simulink model "FrankSensingDiscreteEKF"  (R2025a)
settings: Solver=FixedStepAuto  StartTime=0.0  StopTime=150  FixedStep=.001  RelTol=1e-3
model workspace (MAT data in the model file):
  GPSvehyUpdate = 0
libraries: simulink x1
(part 2 of 2)

== matlab function FrankSensingDiscreteEKF/MATLAB Function1 ==
  data: P output; VYmeas input; X output; VXmeas input; rmeas input; Axmeas input; Xcov input; Ycov input; Ppri input; Xpri input; startflag input; SA input; res output; fk output; Rbiaspri output; Abiaspri output
function [P,X,res,fk,Rbiaspri,Abiaspri] = fcn(VYmeas,VXmeas,rmeas,Axmeas,Xcov,Ycov,Ppri,Xpri, startflag, SA)

a = .3036;
b = .2484;
B = 8.45;
C = 1.6;
D = 73.1580;
E = 1;
Iz = 1;
Mv = 15.7;
delta = SA;
Ts = 0.001;

rvar = .01;
Axvar = .001;


Rk = [Ycov    0    0   0;... 
      0        Xcov    0   0;...
      0        0        rvar    0
      0        0        0       Axvar];  %Measurement noise covariance matrix


Qk = [.02     0      0       0       0       0       0;...
      0      .02      0       0      0       0       0;...
      0      0       .01      0      0       0       0;...
      0      0      0       .01     0       0       0;...
      0      0      0       0       .0001     0       0;...
      0      0      0       0       0       .0001     0;...
      0      0      0       0       0       0       .0001]; % process noise covariance matrix

zk = [VYmeas; VXmeas; rmeas; Axmeas];

% Startup Initialization

if startflag == 0

    Ppredict = [.1     0      0       0       0       0       0;...
      0      .1      0       0      0       0       0;...
      0      0       .1      0      0       0       0;...
      0      0      0       .1     0       0       0;...
      0      0      0       0       .001     0       0;...
      0      0      0       0       0       .001     0;...
      0      0      0       0       0       0       .001];

    
    Xpri = [0.5;-1.9;-.49;0;0.34;-.022;-0.2];
      
else

    Ppredict = Ppri;
end

%Predict:

Vypri = Xpri(1);
Vxpri = Xpri(2);
rpri = Xpri(3);
Psipri = Xpri(4);
Axpri = Xpri(5);
Rbiaspri = Xpri(6);
Abiaspri = Xpri(7);

fk =  LittleF(Abiaspri,Axpri,B,C,D,E,Iz,Mv,Psipri,Rbiaspri,Ts,Vxpri,Vypri,a,b,delta,rpri);

% fk =    [Vypri - Ts*(Vxpri*rpri - (D*sin(C*atan(B*atan((Vypri + b*(Rbiaspri + rpri))/Vxpri) + E*(atan(B*atan((Vypri + b*(Rbiaspri + rpri))/Vxpri)) - B*atan((Vypri + b*(Rbiaspri + rpri))/Vxpri)))) + D*sin(C*atan(E*(atan(B*(delta + atan((Vypri - a*(Rbiaspri + rpri))/Vxpri))) - B*(delta + atan((Vypri - a*(Rbiaspri + rpri))/Vxpri))) + B*(delta + atan((Vypri - a*(Rbiaspri + rpri))/Vxpri))))*cos(delta))/Mv);...
%                                                                                                                                                                                                                                                                                                                                                                      Vxpri + Ts*(Abiaspri + Axpri - Vypri*rpri);...
%     Rbiaspri + rpri - (Ts*(D*b*sin(C*atan(B*atan((Vypri + b*(Rbiaspri + rpri))/Vxpri) + E*(atan(B*atan((Vypri + b*(Rbiaspri + rpri))/Vxpri)) - B*atan((Vypri + b*(Rbiaspri + rpri))/Vxpri)))) - D*a*sin(C*atan(E*(atan(B*(delta + atan((Vypri - a*(Rbiaspri + rpri))/Vxpri))) - B*(delta + atan((Vypri - a*(Rbiaspri + rpri))/Vxpri))) + B*(delta + atan((Vypri - a*(Rbiaspri + rpri))/Vxpri))))*cos(delta)))/Iz;...
%                                                                                                                                                                                                                                                                                                                                                                                   Psipri + Ts*(Rbiaspri + rpri);...
%                                                                                                                                                                                                                                                                                                                                                                                              Abiaspri + Axpri;...
%                                                                                                                                                                                                                                                                                                                                                                                                         Rbiaspri;...
%                                                                                                                                                                                                                                                                                                                                                                                                     Abiaspri];
% 
% 
% 
% 
Fk = BigF(B,C,D,E,Iz,Mv,Rbiaspri,Ts,Vxpri,Vypri,a,b,delta,rpri)

% Fk = [1 - (Ts*((C*D*cos(C*atan(B*atan((Vypri + b*(Rbiaspri + rpri))/Vxpri) + E*(atan(B*atan((Vypri + b*(Rbiaspri + rpri))/Vxpri)) - B*atan((Vypri + b*(Rbiaspri + rpri))/Vxpri))))*(E*(B/(Vxpri*((Vypri + b*(Rbiaspri + rpri))^2/Vxpri^2 + 1)) - B/(Vxpri*((Vypri + b*(Rbiaspri + rpri))^2/Vxpri^2 + 1)*(B^2*atan((Vypri + b*(Rbiaspri + rpri))/Vxpri)^2 + 1))) - B/(Vxpri*((Vypri + b*(Rbiaspri + rpri))^2/Vxpri^2 + 1))))/((B*atan((Vypri + b*(Rbiaspri + rpri))/Vxpri) + E*(atan(B*atan((Vypri + b*(Rbiaspri + rpri))/Vxpri)) - B*atan((Vypri + b*(Rbiaspri + rpri))/Vxpri)))^2 + 1) + (C*D*cos(C*atan(E*(atan(B*(delta + atan((Vypri - a*(Rbiaspri + rpri))/Vxpri))) - B*(delta + atan((Vypri - a*(Rbiaspri + rpri))/Vxpri))) + B*(delta + atan((Vypri - a*(Rbiaspri + rpri))/Vxpri))))*cos(delta)*(E*(B/(Vxpri*((Vypri - a*(Rbiaspri + rpri))^2/Vxpri^2 + 1)) - B/(Vxpri*((Vypri - a*(Rbiaspri + rpri))^2/Vxpri^2 + 1)*(B^2*(delta + atan((Vypri - a*(Rbiaspri + rpri))/Vxpri))^2 + 1))) - B/(Vxpri*((Vypri - a*(Rbiaspri + rpri))^2/Vxpri^2 + 1))))/((E*(atan(B*(delta + atan((Vypri - a*(Rbiaspri + rpri))/Vxpri))) - B*(delta + atan((Vypri - a*(Rbiaspri + rpri))/Vxpri))) + B*(delta + atan((Vypri - a*(Rbiaspri + rpri))/Vxpri)))^2 + 1)))/Mv, -Ts*(rpri - ((C*D*cos(C*atan(B*atan((Vypri + b*(Rbiaspri + rpri))/Vxpri) + E*(atan(B*atan((Vypri + b*(Rbiaspri + rpri))/Vxpri)) - B*atan((Vypri + b*(Rbiaspri + rpri))/Vxpri))))*(E*((B*(Vypri + b*(Rbiaspri + rpri)))/(Vxpri^2*((Vypri + b*(Rbiaspri + rpri))^2/Vxpri^2 + 1)) - (B*(Vypri + b*(Rbiaspri + rpri)))/(Vxpri^2*((Vypri + b*(Rbiaspri + rpri))^2/Vxpri^2 + 1)*(B^2*atan((Vypri + b*(Rbiaspri + rpri))/Vxpri)^2 + 1))) - (B*(Vypri + b*(Rbiaspri + rpri)))/(Vxpri^2*((Vypri + b*(Rbiaspri + rpri))^2/Vxpri^2 + 1))))/((B*atan((Vypri + b*(Rbiaspri + rpri))/Vxpri) + E*(atan(B*atan((Vypri + b*(Rbiaspri + rpri))/Vxpri)) - B*atan((Vypri + b*(Rbiaspri + rpri))/Vxpri)))^2 + 1) + (C*D*cos(C*atan(E*(atan(B*(delta + atan((Vypri - a*(Rbiaspri + rpri))/Vxpri))) - B*(delta + atan((Vypri - a*(Rbiaspri + rpri))/Vxpri))) + B*(delta + atan((Vypri - a*(Rbiaspri + rpri))/Vxpri))))*cos(delta)*(E*((B*(Vypri - a*(Rbiaspri + rpri)))/(Vxpri^2*((Vypri - a*(Rbiaspri + rpri))^2/Vxpri^2 + 1)) - (B*(Vypri - a*(Rbiaspri + rpri)))/(Vxpri^2*((Vypri - a*(Rbiaspri + rpri))^2/Vxpri^2 + 1)*(B^2*(delta + atan((Vypri - a*(Rbiaspri + rpri))/Vxpri))^2 + 1))) - (B*(Vypri - a*(Rbiaspri + rpri)))/(Vxpri^2*((Vypri - a*(Rbiaspri + rpri))^2/Vxpri^2 + 1))))/((E*(atan(B*(delta + atan((Vypri - a*(Rbiaspri + rpri))/Vxpri))) - B*(delta + atan((Vypri - a*(Rbiaspri + rpri))/Vxpri))) + B*(delta + atan((Vypri - a*(Rbiaspri + rpri))/Vxpri)))^2 + 1))/Mv), -Ts*(Vxpri + ((C*D*cos(C*atan(B*atan((Vypri + b*(Rbiaspri + rpri))/Vxpri) + E*(atan(B*atan((Vypri + b*(Rbiaspri + rpri))/Vxpri)) - B*atan((Vypri + b*(Rbiaspri + rpri))/Vxpri))))*(E*((B*b)/(Vxpri*((Vypri + b*(Rbiaspri + rpri))^2/Vxpri^2 + 1)) - (B*b)/(Vxpri*((Vypri + b*(Rbiaspri + rpri))^2/Vxpri^2 + 1)*(B^2*atan((Vypri + b*(Rbiaspri + rpri))/Vxpri)^2 + 1))) - (B*b)/(Vxpri*((Vypri + b*(Rbiaspri + rpri))^2/Vxpri^2 + 1))))/((B*atan((Vypri + b*(Rbiaspri + rpri))/Vxpri) + E*(atan(B*atan((Vypri + b*(Rbiaspri + rpri))/Vxpri)) - B*atan((Vypri + b*(Rbiaspri + rpri))/Vxpri)))^2 + 1) - (C*D*cos(C*atan(E*(atan(B*(delta + atan((Vypri - a*(Rbiaspri + rpri))/Vxpri))) - B*(delta + atan((Vypri - a*(Rbiaspri + rpri))/Vxpri))) + B*(delta + atan((Vypri - a*(Rbiaspri + rpri))/Vxpri))))*cos(delta)*(E*((B*a)/(Vxpri*((Vypri - a*(Rbiaspri + rpri))^2/Vxpri^2 + 1)) - (B*a)/(Vxpri*((Vypri - a*(Rbiaspri + rpri))^2/Vxpri^2 + 1)*(B^2*(delta + atan((Vypri - a*(Rbiaspri + rpri))/Vxpri))^2 + 1))) - (B*a)/(Vxpri*((Vypri - a*(Rbiaspri + rpri))^2/Vxpri^2 + 1))))/((E*(atan(B*(delta + atan((Vypri - a*(Rbiaspri + rpri))/Vxpri))) - B*(delta + atan((Vypri - a*(Rbiaspri + rpri))/Vxpri))) + B*(delta + atan((Vypri - a*(Rbiaspri + rpri))/Vxpri)))^2 + 1))/Mv), 0,  0,        -(Ts*((C*D*cos(C*atan(B*atan((Vypri + b*(Rbiaspri + rpri))/Vxpri) + E*(atan(B*atan((Vypri + b*(Rbiaspri + rpri))/Vxpri)) - B*atan((Vypri + b*(Rbiaspri + rpri))/Vxpri))))*(E*((B*b)/(Vxpri*((Vypri + b*(Rbiaspri + rpri))^2/Vxpri^2 + 1)) - (B*b)/(Vxpri*((Vypri + b*(Rbiaspri + rpri))^2/Vxpri^2 + 1)*(B^2*atan((Vypri + b*(Rbiaspri + rpri))/Vxpri)^2 + 1))) - (B*b)/(Vxpri*((Vypri + b*(Rbiaspri + rpri))^2/Vxpri^2 + 1))))/((B*atan((Vypri + b*(Rbiaspri + rpri))/Vxpri) + E*(atan(B*atan((Vypri + b*(Rbiaspri + rpri))/Vxpri)) - B*atan((Vypri + b*(Rbiaspri + rpri))/Vxpri)))^2 + 1) - (C*D*cos(C*atan(E*(atan(B*(delta + atan((Vypri - a*(Rbiaspri + rpri))/Vxpri))) - B*(delta + atan((Vypri - a*(Rbiaspri + rpri))/Vxpri))) + B*(delta + atan((Vypri - a*(Rbiaspri + rpri))/Vxpri))))*cos(delta)*(E*((B*a)/(Vxpri*((Vypri - a*(Rbiaspri + rpri))^2/Vxpri^2 + 1)) - (B*a)/(Vxpri*((Vypri - a*(Rbiaspri + rpri))^2/Vxpri^2 + 1)*(B^2*(delta + atan((Vypri - a*(Rbiaspri + rpri))/Vxpri))^2 + 1))) - (B*a)/(Vxpri*((Vypri - a*(Rbiaspri + rpri))^2/Vxpri^2 + 1))))/((E*(atan(B*(delta + atan((Vypri - a*(Rbiaspri + rpri))/Vxpri))) - B*(delta + atan((Vypri - a*(Rbiaspri + rpri))/Vxpri))) + B*(delta + atan((Vypri - a*(Rbiaspri + rpri))/Vxpri)))^2 + 1)))/Mv,  0;...
%                                                                                                                                                                                                                                                                                                                                                                                                                                                                                                                                                                                                                                                                                                                                                                                                                                                                                                                                                                                                                                                                                                                                                                                                                                               -Ts*rpri,                                                                                                                                                                                                                                                                                                                                                                                                                                                                                                                                                                                                                                                                                                                                                                                                                                                                                                                                                                                                                                                                                                                                                                                                                                                                                                                                                                                                                                                                  1,                                                                                                                                                                                                                                                                                                                                                                                                                                                                                                                                                                                                                                                                                                                                                                                                                                                                                                                                                                                                                                                                                                                                                                                                                                                                       -Ts*Vypri, 0, Ts,                                                                                                                                                                                                                                                                                                                                                                                                                                                                                                                                                                                                                                                                                                                                                                                                                                                                                                                                                                                                                                                                                                                                                                                                                                                                              0, Ts;...
%     (Ts*((C*D*b*cos(C*atan(B*atan((Vypri + b*(Rbiaspri + rpri))/Vxpri) + E*(atan(B*atan((Vypri + b*(Rbiaspri + rpri))/Vxpri)) - B*atan((Vypri + b*(Rbiaspri + rpri))/Vxpri))))*(E*(B/(Vxpri*((Vypri + b*(Rbiaspri + rpri))^2/Vxpri^2 + 1)) - B/(Vxpri*((Vypri + b*(Rbiaspri + rpri))^2/Vxpri^2 + 1)*(B^2*atan((Vypri + b*(Rbiaspri + rpri))/Vxpri)^2 + 1))) - B/(Vxpri*((Vypri + b*(Rbiaspri + rpri))^2/Vxpri^2 + 1))))/((B*atan((Vypri + b*(Rbiaspri + rpri))/Vxpri) + E*(atan(B*atan((Vypri + b*(Rbiaspri + rpri))/Vxpri)) - B*atan((Vypri + b*(Rbiaspri + rpri))/Vxpri)))^2 + 1) - (C*D*a*cos(C*atan(E*(atan(B*(delta + atan((Vypri - a*(Rbiaspri + rpri))/Vxpri))) - B*(delta + atan((Vypri - a*(Rbiaspri + rpri))/Vxpri))) + B*(delta + atan((Vypri - a*(Rbiaspri + rpri))/Vxpri))))*cos(delta)*(E*(B/(Vxpri*((Vypri - a*(Rbiaspri + rpri))^2/Vxpri^2 + 1)) - B/(Vxpri*((Vypri - a*(Rbiaspri + rpri))^2/Vxpri^2 + 1)*(B^2*(delta + atan((Vypri - a*(Rbiaspri + rpri))/Vxpri))^2 + 1))) - B/(Vxpri*((Vypri - a*(Rbiaspri + rpri))^2/Vxpri^2 + 1))))/((E*(atan(B*(delta + atan((Vypri - a*(Rbiaspri + rpri))/Vxpri))) - B*(delta + atan((Vypri - a*(Rbiaspri + rpri))/Vxpri))) + B*(delta + atan((Vypri - a*(Rbiaspri + rpri))/Vxpri)))^2 + 1)))/Iz,    -(Ts*((C*D*b*cos(C*atan(B*atan((Vypri + b*(Rbiaspri + rpri))/Vxpri) + E*(atan(B*atan((Vypri + b*(Rbiaspri + rpri))/Vxpri)) - B*atan((Vypri + b*(Rbiaspri + rpri))/Vxpri))))*(E*((B*(Vypri + b*(Rbiaspri + rpri)))/(Vxpri^2*((Vypri + b*(Rbiaspri + rpri))^2/Vxpri^2 + 1)) - (B*(Vypri + b*(Rbiaspri + rpri)))/(Vxpri^2*((Vypri + b*(Rbiaspri + rpri))^2/Vxpri^2 + 1)*(B^2*atan((Vypri + b*(Rbiaspri + rpri))/Vxpri)^2 + 1))) - (B*(Vypri + b*(Rbiaspri + rpri)))/(Vxpri^2*((Vypri + b*(Rbiaspri + rpri))^2/Vxpri^2 + 1))))/((B*atan((Vypri + b*(Rbiaspri + rpri))/Vxpri) + E*(atan(B*atan((Vypri + b*(Rbiaspri + rpri))/Vxpri)) - B*atan((Vypri + b*(Rbiaspri + rpri))/Vxpri)))^2 + 1) - (C*D*a*cos(C*atan(E*(atan(B*(delta + atan((Vypri - a*(Rbiaspri + rpri))/Vxpri))) - B*(delta + atan((Vypri - a*(Rbiaspri + rpri))/Vxpri))) + B*(delta + atan((Vypri - a*(Rbiaspri + rpri))/Vxpri))))*cos(delta)*(E*((B*(Vypri - a*(Rbiaspri + rpri)))/(Vxpri^2*((Vypri - a*(Rbiaspri + rpri))^2/Vxpri^2 + 1)) - (B*(Vypri - a*(Rbiaspri + rpri)))/(Vxpri^2*((Vypri - a*(Rbiaspri + rpri))^2/Vxpri^2 + 1)*(B^2*(delta + atan((Vypri - a*(Rbiaspri + rpri))/Vxpri))^2 + 1))) - (B*(Vypri - a*(Rbiaspri + rpri)))/(Vxpri^2*((Vypri - a*(Rbiaspri + rpri))^2/Vxpri^2 + 1))))/((E*(atan(B*(delta + atan((Vypri - a*(Rbiaspri + rpri))/Vxpri))) - B*(delta + atan((Vypri - a*(Rbiaspri + rpri))/Vxpri))) + B*(delta + atan((Vypri - a*(Rbiaspri + rpri))/Vxpri)))^2 + 1)))/Iz,  (Ts*((C*D*b*cos(C*atan(B*atan((Vypri + b*(Rbiaspri + rpri))/Vxpri) + E*(atan(B*atan((Vypri + b*(Rbiaspri + rpri))/Vxpri)) - B*atan((Vypri + b*(Rbiaspri + rpri))/Vxpri))))*(E*((B*b)/(Vxpri*((Vypri + b*(Rbiaspri + rpri))^2/Vxpri^2 + 1)) - (B*b)/(Vxpri*((Vypri + b*(Rbiaspri + rpri))^2/Vxpri^2 + 1)*(B^2*atan((Vypri + b*(Rbiaspri + rpri))/Vxpri)^2 + 1))) - (B*b)/(Vxpri*((Vypri + b*(Rbiaspri + rpri))^2/Vxpri^2 + 1))))/((B*atan((Vypri + b*(Rbiaspri + rpri))/Vxpri) + E*(atan(B*atan((Vypri + b*(Rbiaspri + rpri))/Vxpri)) - B*atan((Vypri + b*(Rbiaspri + rpri))/Vxpri)))^2 + 1) + (C*D*a*cos(C*atan(E*(atan(B*(delta + atan((Vypri - a*(Rbiaspri + rpri))/Vxpri))) - B*(delta + atan((Vypri - a*(Rbiaspri + rpri))/Vxpri))) + B*(delta + atan((Vypri - a*(Rbiaspri + rpri))/Vxpri))))*cos(delta)*(E*((B*a)/(Vxpri*((Vypri - a*(Rbiaspri + rpri))^2/Vxpri^2 + 1)) - (B*a)/(Vxpri*((Vypri - a*(Rbiaspri + rpri))^2/Vxpri^2 + 1)*(B^2*(delta + atan((Vypri - a*(Rbiaspri + rpri))/Vxpri))^2 + 1))) - (B*a)/(Vxpri*((Vypri - a*(Rbiaspri + rpri))^2/Vxpri^2 + 1))))/((E*(atan(B*(delta + atan((Vypri - a*(Rbiaspri + rpri))/Vxpri))) - B*(delta + atan((Vypri - a*(Rbiaspri + rpri))/Vxpri))) + B*(delta + atan((Vypri - a*(Rbiaspri + rpri))/Vxpri)))^2 + 1)))/Iz + 1, 0,  0, (Ts*((C*D*b*cos(C*atan(B*atan((Vypri + b*(Rbiaspri + rpri))/Vxpri) + E*(atan(B*atan((Vypri + b*(Rbiaspri + rpri))/Vxpri)) - B*atan((Vypri + b*(Rbiaspri + rpri))/Vxpri))))*(E*((B*b)/(Vxpri*((Vypri + b*(Rbiaspri + rpri))^2/Vxpri^2 + 1)) - (B*b)/(Vxpri*((Vypri + b*(Rbiaspri + rpri))^2/Vxpri^2 + 1)*(B^2*atan((Vypri + b*(Rbiaspri + rpri))/Vxpri)^2 + 1))) - (B*b)/(Vxpri*((Vypri + b*(Rbiaspri + rpri))^2/Vxpri^2 + 1))))/((B*atan((Vypri + b*(Rbiaspri + rpri))/Vxpri) + E*(atan(B*atan((Vypri + b*(Rbiaspri + rpri))/Vxpri)) - B*atan((Vypri + b*(Rbiaspri + rpri))/Vxpri)))^2 + 1) + (C*D*a*cos(C*atan(E*(atan(B*(delta + atan((Vypri - a*(Rbiaspri + rpri))/Vxpri))) - B*(delta + atan((Vypri - a*(Rbiaspri + rpri))/Vxpri))) + B*(delta + atan((Vypri - a*(Rbiaspri + rpri))/Vxpri))))*cos(delta)*(E*((B*a)/(Vxpri*((Vypri - a*(Rbiaspri + rpri))^2/Vxpri^2 + 1)) - (B*a)/(Vxpri*((Vypri - a*(Rbiaspri + rpri))^2/Vxpri^2 + 1)*(B^2*(delta + atan((Vypri - a*(Rbiaspri + rpri))/Vxpri))^2 + 1))) - (B*a)/(Vxpri*((Vypri - a*(Rbiaspri + rpri))^2/Vxpri^2 + 1))))/((E*(atan(B*(delta + atan((Vypri - a*(Rbiaspri + rpri))/Vxpri))) - B*(delta + atan((Vypri - a*(Rbiaspri + rpri))/Vxpri))) + B*(delta + atan((Vypri - a*(Rbiaspri + rpri))/Vxpri)))^2 + 1)))/Iz + 1,  0;...
%                                                                                                                                                                                                                                                                                                                                                                                                                                                                                                                                                                                                                                                                                                                                                                                                                                                                                                                                                                                                                                                                                                                                                                                                                                                      0,                                                                                                                                                                                                                                                                                                                                                                                                                                                                                                                                                                                                                                                                                                                                                                                                                                                                                                                                                                                                                                                                                                                                                                                                                                                                                                                                                                                                                                                                  0,                                                                                                                                                                                                                                                                                                                                                                                                                                                                                                                                                                                                                                                                                                                                                                                                                                                                                                                                                                                                                                                                                                                                                                                                                                                                              Ts, 1,  0,                                                                                                                                                                                                                                                                                                                                                                                                                                                                                                                                                                                                                                                                                                                                                                                                                                                                                                                                                                                                                                                                                                                                                                                                                                                                             Ts,  0;...
%                                                                                                                                                                                                                                                                                                                                                                                                                                                                                                                                                                                                                                                                                                                                                                                                                                                                                                                                                                                                                                                                                                                                                                                                                                                      0,                                                                                                                                                                                                                                                                                                                                                                                                                                                                                                                                                                                                                                                                                                                                                                                                                                                                                                                                                                                                                                                                                                                                                                                                                                                                                                                                                                                                                                                                  0,                                                                                                                                                                                                                                                                                                                                                                                                                                                                                                                                                                                                                                                                                                                                                                                                                                                                                                                                                                                                                                                                                                                                                                                                                                                                               0, 0,  1,                                                                                                                                                                                                                                                                                                                                                                                                                                                                                                                                                                                                                                                                                                                                                                                                                                                                                                                                                                                                                                                                                                                                                                                                                                                                              0,  1;...
%                                                                                                                                                                                                                                                                                                                                                                                                                                                                                                                                                                                                                                                                                                                                                                                                                                                                                                                                                                                                                                                                                                                                                                                                                                                      0,                                                                                                                                                                                                                                                                                                                                                                                                                                                                                                                                                                                                                                                                                                                                                                                                                                                                                                                                                                                                                                                                                                                                                                                                                                                                                                                                                                                                                                                                  0,                                                                                                                                                                                                                                                                                                                                                                                                                                                                                                                                                                                                                                                                                                                                                                                                                                                                                                                                                                                                                                                                                                                                                                                                                                                                               0, 0,  0,                                                                                                                                                                                                                                                                                                                                                                                                                                                                                                                                                                                                                                                                                                                                                                                                                                                                                                                                                                                                                                                                                                                                                                                                                                                                              1,  0;...
%                                                                                                                                                                                                                                                                                                                                                                                                                                                                                                                                                                                                                                                                                                                                                                                                                                                                                                                                                                                                                                                                                                                                                                                                                                                      0,                                                                                                                                                                                                                                                                                                                                                                                                                                                                                                                                                                                                                                                                                                                                                                                                                                                                                                                                                                                                                                                                                                                                                                                                                                                                                                                                                                                                                                                                  0,                                                                                                                                                                                                                                                                                                                                                                                                                                                                                                                                                                                                                                                                                                                                                                                                                                                                                                                                                                                                                                                                                                                                                                                                                                                                               0, 0,  0,                                                                                                                                                                                                                                                                                                                                                                                                                                                                                                                                                                                                                                                                                                                                                                                                                                                                                                                                                                                                                                                                                                                                                                                                                                                                              0,  1];
% 

Ppost = Fk*Ppredict*Fk'+Qk;

hk = [fk(2)*sin(fk(4))+fk(1)*cos(fk(4));fk(2)*cos(fk(4))-fk(1)*sin(fk(4));fk(3);fk(5)];

Hk = [cos(fk(4))   sin(fk(4))     0   fk(2)*cos(fk(4))-fk(1)*sin(fk(4))     0       0       0;...
      -sin(fk(4))  cos(fk(4))     0   -fk(1)*cos(fk(4))-fk(2)*sin(fk(4))    0       0       0;...
      0             0               1   0                                       0       0       0;...
      0             0               0   0                                       1       0       0];



%Update:

res = zk-hk;
Sk = Hk*Ppost*Hk'+Rk;
Kk = Ppost*Hk'*inv(Sk);
X = fk+Kk*res;
P = (eye(7,7)-Kk*Hk)*Ppost
